simulink model "manning_test_merge_linear"  (R2022b)
settings: Solver=VariableStepAuto  StartTime=0.0  StopTime=5*34416  RelTol=1e-3
undefined symbols (not defined in the file or in its folder): gain, yd_ds
settings Model: Creator=chuan  LastModifiedBy=chuan

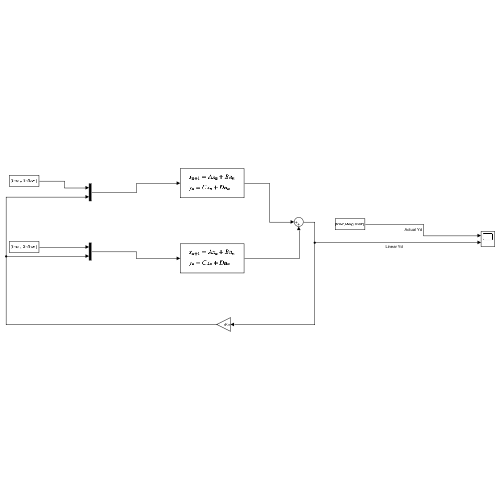
[thumbnail: Simulink's stored preview of the top-level diagram]
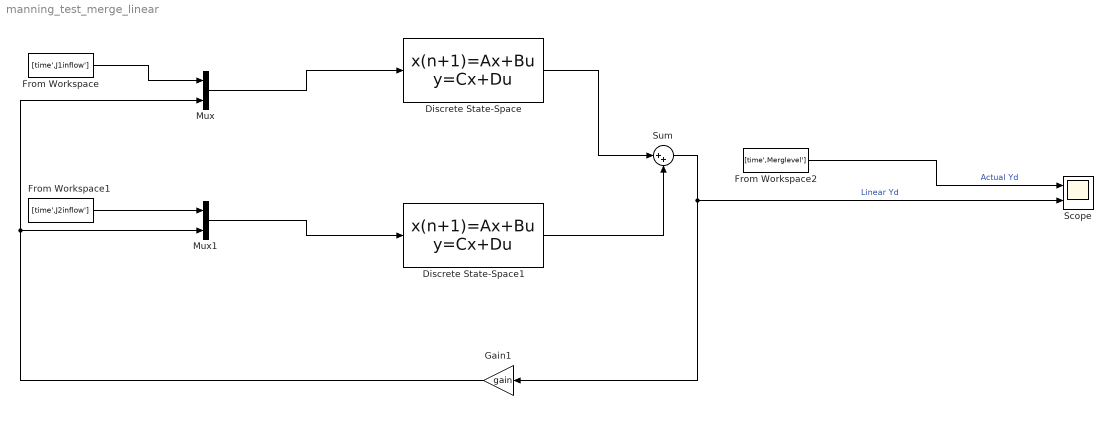
== system manning_test_merge_linear ==
  Discrete State-Space : DiscreteStateSpace  A=yd_ds{1}.A  B=yd_ds{1}.B  C=yd_ds{1}.C  D=yd_ds{1}.D  SampleTime=yd_ds{1}.Ts
  Discrete State-Space1 : DiscreteStateSpace  A=yd_ds{2}.A  B=yd_ds{2}.B  C=yd_ds{2}.C  D=yd_ds{2}.D  SampleTime=yd_ds{2}.Ts
  From Workspace : FromWorkspace  VariableName=[time',J1inflow']
  From Workspace1 : FromWorkspace  VariableName=[time',J2inflow']
  From Workspace2 : FromWorkspace  VariableName=[time',Merglevel']
  Gain1 : Gain  Gain=gain
  Mux : Mux  Inputs=2
  Mux1 : Mux  Inputs=2
  Scope : Scope  NumInputPorts=2
  Sum : Sum  Inputs=|++
  wires:
  Mux/1 -> Discrete State-Space/1
  From Workspace/1 -> Mux/1
  From Workspace2/1 -> Scope/1  "Actual Yd"
  From Workspace1/1 -> Mux1/1
  Mux1/1 -> Discrete State-Space1/1
  Discrete State-Space1/1 -> Sum/2
  Discrete State-Space/1 -> Sum/1
  Sum/1 -> Gain1/1, Scope/2  "Linear Yd"
  Gain1/1 -> Mux1/2, Mux/2
